simulink model "sampleModel1737"  (R2023a)
settings: Solver=VariableStepAuto  StartTime=0.0  StopTime=10.0  RelTol=1e-3
libraries: hdlsllib x5, simulink x3
settings Model: Creator=user1  LastModifiedBy=user1

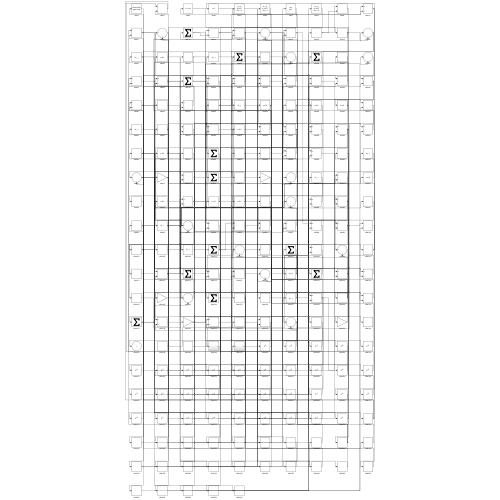
[thumbnail: Simulink's stored preview of the top-level diagram]
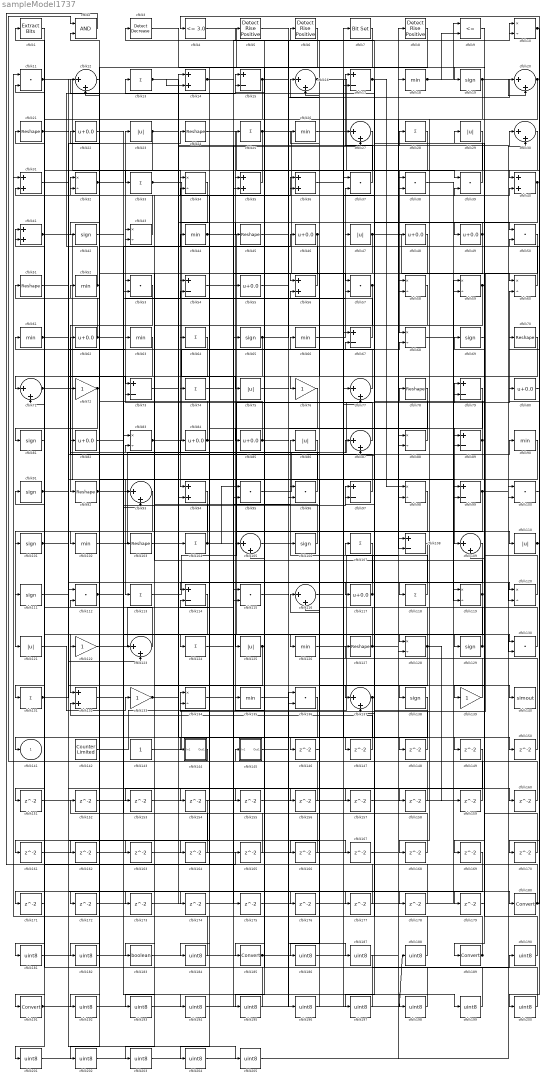
== system sampleModel1737 ==
  cfblk1 : simulink/Logic and Bit Operations/Extract Bits  bitsToExtract=Upper half  numBits=8  bitIdxRange=[0 7]  outScalingMode=Preserve fixed-point scaling
      settings: LibrarySourceBlock=|
      | hdlsllib/Logic and Bit
      | Operations/Extract Bits
  cfblk{10,32,34,43,58..60,68,83,88,98,119..120,128,134} (15 alike) : Product  Inputs=*/  RndMeth=Zero  SaturateOnIntegerOverflow=on
  cfblk{11,37..39,50,53,57,95..96,100,112,115,130,136} (14 alike) : DotProduct  OutDataTypeStr=Inherit: Inherit via internal rule
  cfblk{19,42,65,69,81,91,101,106,111,129,138} (11 alike) : Signum
  cfblk{18,26,44,52,61,63,66,90,102,126,135} (11 alike) : MinMax
  cfblk{21,24,45,51,70,78,92,103,127} (9 alike) : Reshape
  cfblk{13,25,28,33,64,74,104,107,113,118,124,131} (12 alike) : Sum  Inputs=+
  cfblk{12,16,20,27,30,71,77,87,93,105,109,116,123,137} (14 alike) : Sum  Inputs=|++
  cfblk{15,17,54,67,73,79,89,97,99,108,114} (11 alike) : Sum  Inputs=+-
  cfblk{23,29,47,75,86,110,121,125} (8 alike) : Abs  SaturateOnIntegerOverflow=off
  cfblk{22,46,48..49,55,62,80,82,84..85,117} (11 alike) : Bias  Bias=0.0  SaturateOnIntegerOverflow=off
  cfblk{72,76,122,133,139} (5 alike) : Gain
  cfblk{14,31,35..36,40..41,56,94,132} (9 alike) : Sum
  cfblk140 : ToWorkspace  VariableName=simout  SaveFormat=Timeseries  SampleTime=-1
  cfblk142 : hdlsllib/Sources/Counter Limited  uplimit=7  tsamp=-1
  cfblk143 : Constant  SampleTime=-1
  cfblk144 : Subsystem
      settings: LibrarySourceBlock=|
      | hdlsllib/Ports &
      | Subsystems/Subsystem
  cfblk145 : Subsystem
      settings: LibrarySourceBlock=|
      | hdlsllib/Ports &
      | Subsystems/Subsystem
  cfblk{146..179} (34 alike) : Delay  SampleTime=1
  cfblk{180,185,189,191} (4 alike) : DataTypeConversion  SaturateOnIntegerOverflow=off  RndMeth=Floor
  cfblk{181..182,184,186..188,190,192..205} (21 alike) : DataTypeConversion  OutDataTypeStr=uint8  SaturateOnIntegerOverflow=off  RndMeth=Floor
  cfblk183 : DataTypeConversion  OutDataTypeStr=boolean  SaturateOnIntegerOverflow=off  RndMeth=Floor
  cfblk2 : Logic  AllPortsSameDT=off  OutDataTypeStr=boolean
  cfblk3 : simulink/Logic and Bit Operations/Detect Decrease  vinit=0.0  OutDataTypeStr=boolean
      settings: LibrarySourceBlock=|
      | hdlsllib/Logic and Bit
      | Operations/Detect
      | Decrease
  cfblk4 : hdlsllib/Logic and Bit Operations/Compare To Constant  relop=<=  const=3.0  OutDataTypeStr=boolean
  cfblk5 : hdlsllib/Logic and Bit Operations/Detect Rise Positive  vinit=0  OutDataTypeStr=boolean
  cfblk6 : hdlsllib/Logic and Bit Operations/Detect Rise Positive  vinit=0  OutDataTypeStr=boolean
  cfblk7 : simulink/Logic and Bit Operations/Bit Set  iBit=0
      settings: LibrarySourceBlock=|
      | hdlsllib/Logic and Bit
      | Operations/Bit Set
  cfblk8 : hdlsllib/Logic and Bit Operations/Detect Rise Positive  vinit=0  OutDataTypeStr=boolean
  cfblk9 : RelationalOperator  Operator=<=  OutDataTypeStr=boolean  InputSameDT=off
  cfblk141 : Outport  VectorParamsAs1DForOutWhenUnconnected=off
  wires:
  cfblk44/1 -> cfblk126/1, cfblk50/1
  cfblk89/1 -> cfblk32/1, cfblk156/1, cfblk157/1
  cfblk52/1 -> cfblk15/1, cfblk122/1
  cfblk4/1 -> cfblk139/1
  cfblk67/1 -> cfblk23/1
  cfblk50/1 -> cfblk134/1
  cfblk34/1 -> cfblk94/1
  cfblk125/1 -> cfblk153/1, cfblk195/1
  cfblk24/1 -> cfblk68/1
  cfblk80/1 -> cfblk4/1
  cfblk54/1 -> cfblk110/1
  cfblk66/1 -> cfblk37/2
  cfblk62/1 -> cfblk11/2, cfblk93/2, cfblk160/1
  cfblk29/1 -> cfblk33/1
  cfblk16/1 -> cfblk39/1, cfblk99/1
  cfblk117/1 -> cfblk107/1, cfblk114/1
  cfblk53/1 -> cfblk92/1
  cfblk105/1 -> cfblk86/1
  cfblk79/1 -> cfblk109/1
  cfblk106/1 -> cfblk43/1
  cfblk3/1 -> cfblk19/1
  cfblk87/1 -> cfblk53/1
  cfblk41/1 -> cfblk113/1, cfblk177/1
  cfblk86/1 -> cfblk102/1
  cfblk101/1 -> cfblk90/1, cfblk205/1
  cfblk71/1 -> cfblk104/1, cfblk120/1, cfblk167/1
  cfblk94/1 -> cfblk121/1
  cfblk25/1 -> cfblk57/1, cfblk144/1(In1)
  cfblk114/1 -> cfblk132/1
  cfblk104/1 -> cfblk31/2, cfblk96/1, cfblk95/1
  cfblk118/1 -> cfblk106/1
  cfblk137/1 -> cfblk47/1, cfblk174/1
  cfblk130/1 -> cfblk43/2
  cfblk88/1 -> cfblk13/1
  cfblk97/1 -> cfblk62/1
  cfblk143/1 -> cfblk25/1
  cfblk33/1 -> cfblk75/1, cfblk99/2
  cfblk15/1 -> cfblk89/2, cfblk151/1
  cfblk121/1 -> cfblk133/1
  cfblk126/1 -> cfblk8/1
  cfblk47/1 -> cfblk60/1, cfblk173/1
  cfblk77/1 -> cfblk41/1
  cfblk11/1 -> cfblk64/1, cfblk93/1
  cfblk91/1 -> cfblk24/1, cfblk140/1
  cfblk60/1 -> cfblk12/1
  cfblk1/1 -> cfblk131/1
  cfblk13/1 -> cfblk14/2, cfblk137/1
  cfblk35/1 -> cfblk34/1
  cfblk103/1 -> cfblk128/1
  cfblk61/1 -> cfblk119/2, cfblk120/2, cfblk154/1
  cfblk43/1 -> cfblk21/1
  cfblk142/1 -> cfblk38/1
  cfblk21/1 -> cfblk71/1, cfblk73/1
  cfblk95/1 -> cfblk60/2
  cfblk74/1 -> cfblk30/1
  cfblk112/1 -> cfblk97/1, cfblk57/2
  cfblk39/1 -> cfblk3/1
  cfblk113/1 -> cfblk79/1
  cfblk127/1 -> cfblk44/1, cfblk39/2
  cfblk22/1 -> cfblk53/2
  cfblk133/1 -> cfblk28/1, cfblk36/1
  cfblk68/1 -> cfblk119/1
  cfblk31/1 -> cfblk112/1
  cfblk14/1 -> cfblk56/1, cfblk10/2
  cfblk28/1 -> cfblk117/1
  cfblk20/1 -> cfblk95/2, cfblk168/1
  cfblk132/1 -> cfblk46/1
  cfblk136/1 -> cfblk191/1
  cfblk48/1 -> cfblk72/1
  cfblk49/1 -> cfblk76/1, cfblk48/1
  cfblk37/1 -> cfblk17/1
  cfblk36/1 -> cfblk118/1
  cfblk38/1 -> cfblk89/1
  cfblk84/1 -> cfblk52/1, cfblk150/1
  cfblk30/1 -> cfblk81/1
  cfblk102/1 -> cfblk59/1
  cfblk83/1 -> cfblk68/2, cfblk27/2
  cfblk115/1 -> cfblk180/1
  cfblk12/1 -> cfblk42/1
  cfblk129/1 -> cfblk83/2, cfblk124/1, cfblk82/1
  cfblk128/1 -> cfblk36/2, cfblk158/1, cfblk159/1, cfblk186/1
  cfblk40/1 -> cfblk49/1, cfblk137/2
  cfblk131/1 -> cfblk63/1, cfblk123/2
  cfblk90/1 -> cfblk105/2
  cfblk59/1 -> cfblk129/1, cfblk85/1, cfblk96/2
  cfblk6/1 -> cfblk185/1
  cfblk99/1 -> cfblk111/1, cfblk30/2
  cfblk116/1 -> cfblk77/2
  cfblk57/1 -> cfblk163/1, cfblk164/1
  cfblk32/1 -> cfblk125/1, cfblk199/1
  cfblk85/1 -> cfblk22/1, cfblk130/2
  cfblk122/1 -> cfblk65/1
  cfblk42/1 -> cfblk138/1
  cfblk10/1 -> cfblk40/1, cfblk170/1
  cfblk92/1 -> cfblk84/1, cfblk40/2, cfblk67/1
  cfblk65/1 -> cfblk103/1, cfblk10/1
  cfblk19/1 -> cfblk108/2, cfblk20/2
  cfblk110/1 -> cfblk80/1, cfblk50/2
  cfblk46/1 -> cfblk16/2, cfblk183/1
  cfblk45/1 -> cfblk130/1
  cfblk56/1 -> cfblk35/1
  cfblk70/1 -> cfblk101/1
  cfblk82/1 -> cfblk123/1
  cfblk23/1 -> cfblk45/1, cfblk71/2
  cfblk139/1 -> cfblk26/1
  cfblk27/1 -> cfblk54/1
  cfblk123/1 -> cfblk51/1
  cfblk69/1 -> cfblk189/1
  cfblk72/1 -> cfblk171/1, cfblk172/1
  cfblk119/1 -> cfblk141/1, cfblk73/2
  cfblk120/1 -> cfblk78/1
  cfblk17/1 -> cfblk98/1, cfblk147/1
  cfblk64/1 -> cfblk74/1
  cfblk18/1 -> cfblk9/1, cfblk9/2
  cfblk144/1(Out1) -> cfblk2/1
  cfblk108/1 -> cfblk116/2
  cfblk134/1 -> cfblk87/1
  cfblk96/1 -> cfblk2/2
  cfblk55/1 -> cfblk20/1
  cfblk107/1 -> cfblk146/1
  cfblk146/1 -> cfblk56/2
  cfblk147/1 -> cfblk132/2
  cfblk73/1 -> cfblk148/1
  cfblk148/1 -> cfblk105/1
  cfblk26/1 -> cfblk149/1
  cfblk150/1 -> cfblk16/1
  cfblk151/1 -> cfblk77/1
  cfblk153/1 -> cfblk59/2
  cfblk78/1 -> cfblk155/1
  cfblk155/1 -> cfblk15/2
  cfblk156/1 -> cfblk134/2
  cfblk157/1 -> cfblk87/2
  cfblk158/1 -> cfblk34/2
  cfblk159/1 -> cfblk54/2
  cfblk160/1 -> cfblk31/1
  cfblk81/1 -> cfblk161/1
  cfblk161/1 -> cfblk108/1
  cfblk93/1 -> cfblk162/1
  cfblk162/1 -> cfblk17/2
  cfblk163/1 -> cfblk128/2
  cfblk164/1 -> cfblk112/2
  cfblk2/1 -> cfblk165/1
  cfblk165/1 -> cfblk14/1
  cfblk138/1 -> cfblk166/1
  cfblk166/1 -> cfblk12/2
  cfblk167/1 -> cfblk98/2
  cfblk168/1 -> cfblk83/1
  cfblk9/1 -> cfblk169/1
  cfblk170/1 -> cfblk109/2
  cfblk171/1 -> cfblk41/2
  cfblk172/1 -> cfblk27/1
  cfblk173/1 -> cfblk94/2
  cfblk174/1 -> cfblk79/2
  cfblk124/1 -> cfblk175/1
  cfblk175/1 -> cfblk88/2
  cfblk51/1 -> cfblk176/1
  cfblk176/1 -> cfblk116/1
  cfblk177/1 -> cfblk114/2
  cfblk111/1 -> cfblk178/1
  cfblk178/1 -> cfblk1/1
  cfblk75/1 -> cfblk179/1
  cfblk179/1 -> cfblk29/1
  cfblk180/1 -> cfblk67/2, cfblk91/1, cfblk70/1
  cfblk169/1 -> cfblk181/1
  cfblk181/1 -> cfblk115/1
  cfblk98/1 -> cfblk182/1
  cfblk182/1 -> cfblk115/2
  cfblk183/1 -> cfblk7/1
  cfblk7/1 -> cfblk184/1
  cfblk184/1 -> cfblk32/2
  cfblk185/1 -> cfblk18/1, cfblk55/1
  cfblk186/1 -> cfblk6/1
  cfblk135/1 -> cfblk187/1
  cfblk188/1 -> cfblk135/1
  cfblk189/1 -> cfblk11/1, cfblk97/2, cfblk127/1
  cfblk187/1 -> cfblk190/1
  cfblk190/1 -> cfblk69/1
  cfblk191/1 -> cfblk188/1, cfblk35/2
  cfblk63/1 -> cfblk192/1
  cfblk192/1 -> cfblk136/1
  cfblk149/1 -> cfblk193/1
  cfblk193/1 -> cfblk136/2
  cfblk152/1 -> cfblk194/1
  cfblk194/1 -> cfblk37/1
  cfblk195/1 -> cfblk152/1
  cfblk5/1 -> cfblk196/1
  cfblk196/1 -> cfblk66/1
  cfblk109/1 -> cfblk197/1
  cfblk197/1 -> cfblk5/1
  cfblk145/1(Out1) -> cfblk198/1
  cfblk198/1 -> cfblk61/1
  cfblk199/1 -> cfblk145/1(In1)
  cfblk100/1 -> cfblk200/1
  cfblk200/1 -> cfblk88/1
  cfblk154/1 -> cfblk201/1
  cfblk201/1 -> cfblk100/1
  cfblk8/1 -> cfblk202/1
  cfblk202/1 -> cfblk100/2
  cfblk58/1 -> cfblk203/1
  cfblk203/1 -> cfblk38/2
  cfblk76/1 -> cfblk204/1
  cfblk204/1 -> cfblk58/1
  cfblk205/1 -> cfblk58/2

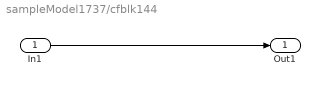
== system sampleModel1737/cfblk144 ==
  In1 : Inport
  Out1 : Outport
  wires:
  In1/1 -> Out1/1

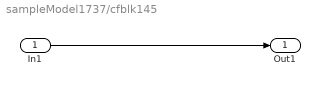
== system sampleModel1737/cfblk145 ==
  In1 : Inport
  Out1 : Outport
  wires:
  In1/1 -> Out1/1
